simulink model "FIG_1_2021_JEVG"  (R2021a)
settings: Solver=VariableStepAuto  StartTime=0.0  StopTime=10.0  RelTol=1e-3
settings Model: Creator=mluser  LastModifiedBy=user
settings DebuggingCC: UnconnectedInputMsg=none  UnconnectedOutputMsg=none  UnconnectedLineMsg=none
settings ModelReferenceCC: EnableRefExpFcnMdlSchedulingChecks=off
settings RTWCC: Description=Generic Real-Time Target  DLArmComputeVersion=20.02.1

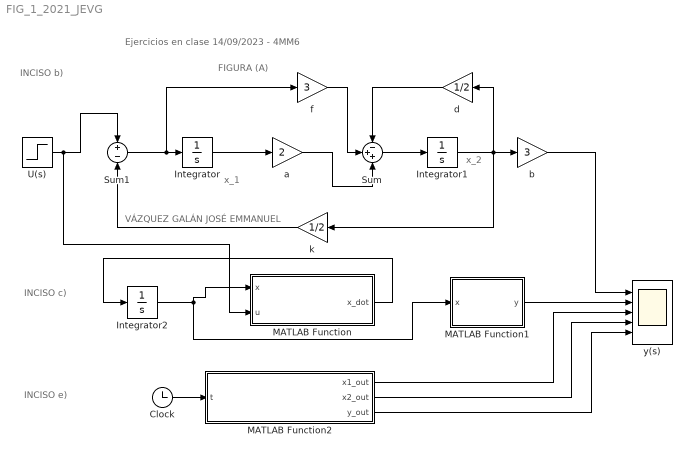
== system FIG_1_2021_JEVG ==
  note: Ejercicios en clase 14/09/2023 - 4MM6
  note: INCISO b)
  note: x_1
  note: VÁZQUEZ GALÁN JOSÉ EMMANUEL
  note: x_2
  note: FIGURA (A)
  note: INCISO c)
  note: INCISO e)
  Clock : Clock
  Integrator : Integrator
  Integrator1 : Integrator
  Integrator2 : Integrator
  MATLAB Function : MATLAB Function  TreatAsAtomicUnit=on
  MATLAB Function1 : MATLAB Function  TreatAsAtomicUnit=on
  MATLAB Function2 : MATLAB Function  TreatAsAtomicUnit=on
  Sum : Sum  Inputs=-++
  Sum1 : Sum  Inputs=+-
  U(s) : Step  SampleTime=0
  a : Gain  Gain=2
  b : Gain  Gain=3
  d : Gain  Gain=1/2
  f : Gain  Gain=3
  k : Gain  Gain=1/2
  y(s) : Scope  NumInputPorts=5
  wires:
  Integrator/1 -> a/1
  a/1 -> Sum/3
  f/1 -> Sum/2
  U(s)/1 -> MATLAB Function/2(u), Sum1/1
  k/1 -> Sum1/2
  Sum/1 -> Integrator1/1
  Integrator1/1 -> k/1, d/1, b/1
  b/1 -> y(s)/1
  d/1 -> Sum/1
  Sum1/1 -> f/1, Integrator/1
  MATLAB Function/1(x_dot) -> Integrator2/1
  MATLAB Function1/1(y) -> y(s)/2
  Integrator2/1 -> MATLAB Function/1(x), MATLAB Function1/1(x)
  Clock/1 -> MATLAB Function2/1(t)
  MATLAB Function2/1(x1_out) -> y(s)/3
  MATLAB Function2/2(x2_out) -> y(s)/4
  MATLAB Function2/3(y_out) -> y(s)/5

== matlab function FIG_1_2021_JEVG/MATLAB Function ==
  data: x input size=[2, 1]; u input size=[1, 1]; x_dot output size=[2, 1]
function x_dot = stateSpaceSystem(x, u)
    % Definición de constantes (asumiendo valores para k, f, d, y a)
    a = 2;
    d = 1/2;
    k = 1/2;
    f = 3; 
    
    % Matrices A y B
    A = [0, -k; a, -(f*k+d)];
    B = [1; f];

    % Sistema en espacio de estado
    x_dot = A*x + B*u;
end

== matlab function FIG_1_2021_JEVG/MATLAB Function2 ==
  data: x1_out output; x2_out output; t input; y_out output
function [x1_out, x2_out, y_out] = stateResponse(t)
    if t < 1
        x1_out = 0;
        x2_out = 0;
        y_out = 0;
    else
        x1_out = x1_func(t-1);
        x2_out = x2_func(t-1);
        y_out = y_func(t-1);
    end
end

== matlab function FIG_1_2021_JEVG/MATLAB Function1 ==
  data: x input; y output
function y = outputFunction(x)
    % Definición de constantes (asumiendo un valor para b)
    b = 3;

    % Matriz C
    C = [0, b];

    % Cálculo de la salida
    y = C*x;
end
